simulink model "COSTEP"  (R2024b)
settings: Solver=FixedStepAuto  StartTime=0.0  StopTime=25  FixedStep=1/3600  RelTol=1e-3
model workspace (MAT data in the model file):
  AD : Simulink.Parameter (value not decoded)
  AG : Simulink.Parameter (value not decoded)
  AH : Simulink.Parameter (value not decoded)
  AV : Simulink.Parameter (value not decoded)
  AVP : Simulink.Parameter (value not decoded)
  BCHL : Simulink.Parameter (value not decoded)
  BCHV : Simulink.Parameter (value not decoded)
  BD : Simulink.Parameter (value not decoded)
  BDIST : Simulink.Parameter (value not decoded)
  BG : Simulink.Parameter (value not decoded)
  BH : Simulink.Parameter (value not decoded)
  BVP : Simulink.Parameter (value not decoded)
  CD : Simulink.Parameter (value not decoded)
  CDIST : Simulink.Parameter (value not decoded)
  CG : Simulink.Parameter (value not decoded)
  CH : Simulink.Parameter (value not decoded)
  CVP : Simulink.Parameter (value not decoded)
  DDIST : Simulink.Parameter (value not decoded)
  DIST_CONST : Simulink.Parameter (value not decoded)
  ISV : Simulink.Parameter (value not decoded)
  TLAST : Simulink.Parameter (value not decoded)
  TNEXT : Simulink.Parameter (value not decoded)
  XMW : Simulink.Parameter (value not decoded)
  XNS : Simulink.Parameter (value not decoded)
  XNS2 : Simulink.Parameter (value not decoded)
  XNS3 : Simulink.Parameter (value not decoded)
  XNSADD : Simulink.Parameter (value not decoded)
  XNSE : Simulink.Parameter (value not decoded)
symbols that are objects in the model workspace (value not decoded): AD, AG, AH, AV, AVP, BD, BG, BH, BVP, CD, CG, CH, CVP, XMW, XNS, XNS2, XNS3, XNSE
undefined symbols (not defined in the file or in its folder): magnitude, msgbox, SETPT, XMEAS, XMV
libraries: mylib x381, dspindex x31
(part 9 of 12)

== system COSTEP/Stream Measurements/Subsystem6/Product stream/Temperature measurement in C ==
  XMEAS in celsius : Inport
  SMEAST : Outport
  wires:
  XMEAS in celsius/1 -> SMEAST/1  "SMEAST"

== system COSTEP/Stream Measurements/Subsystem6/Purge stream/Composition measurement mol% ==
  XMEAS : Inport
  Bus Creator : BusCreator  Inputs=8
  Bus Selector : BusSelector  OutputSignals=XMEAS(29),XMEAS(30),XMEAS(31),XMEAS(32),XMEAS(33),XMEAS(34),XMEAS(35),XMEAS(36)
  SMEASX(9) : Outport
  wires:
  Bus Selector/4 -> Bus Creator/4  "<XMEAS(32)>"
  Bus Selector/5 -> Bus Creator/5  "<XMEAS(33)>"
  Bus Selector/6 -> Bus Creator/6  "<XMEAS(34)>"
  Bus Selector/7 -> Bus Creator/7  "<XMEAS(35)>"
  Bus Selector/8 -> Bus Creator/8  "<XMEAS(36)>"
  Bus Selector/3 -> Bus Creator/3  "<XMEAS(31)>"
  XMEAS/1 -> Bus Selector/1
  Bus Selector/2 -> Bus Creator/2  "<XMEAS(30)>"
  Bus Selector/1 -> Bus Creator/1  "<XMEAS(29)>"
  Bus Creator/1 -> SMEASX(9)/1  "SMEASX"

== system COSTEP/Stream Measurements/Subsystem6/Purge stream/Flow measurement in kg//h ==
  XMEAS in kscmh : Inport
  XST : Inport  Port=2
  " " : Constant  Value=35.3145
  "  " : Constant  Value=0.359
  Convert from lb/h to kg/h : Constant  Value=0.454
  Product : Product  Inputs=3
  XMWS Molecular weight of Stream lb/lb-mol : Subsystem
  lb-mol/h : Product  Inputs=**/
  "SMEASF(9) " : Outport  VectorParamsAs1DForOutWhenUnconnected=off
  wires:
  " "/1 -> lb-mol/h/2
  "  "/1 -> lb-mol/h/3
  XMEAS in kscmh/1 -> lb-mol/h/1
  Convert from lb/h to kg/h/1 -> Product/3
  XST/1 -> XMWS Molecular weight of Stream lb/lb-mol/1(XST)
  lb-mol/h/1 -> Product/2
  XMWS Molecular weight of Stream lb/lb-mol/1(XMWS) -> Product/1
  Product/1 -> "SMEASF(9) "/1

== system COSTEP/Stream Measurements/Subsystem6/Purge stream/Pressure measurement in kPa ==
  XMNSE : Inport
  " kPa" : Constant  Value=101.325
  Add : Sum
  SMEASP(9) : Outport  VectorParamsAs1DForOutWhenUnconnected=off
  wires:
  Add/1 -> SMEASP(9)/1  "SMEASP"
  " kPa"/1 -> Add/1
  XMNSE/1 -> Add/2

== system COSTEP/Stream Measurements/Subsystem6/Purge stream/Temperature measurement in C ==
  XMEAS in celsius : Inport
  SMEAST(9) : Outport
  wires:
  XMEAS in celsius/1 -> SMEAST(9)/1  "SMEAST"

== system COSTEP/Stream Measurements/Subsystem6/RCIn/Flow measurement in kg//h ==
  XMNSE : Inport
  F in gpm : Inport  Port=2
  Add : Sum
  Product : Product
  Product1 : Product
  gpm to lb/h : Constant  Value=500.72
  kg/kmol : Constant  Value=18.02
  kmol : Constant  Value=0.45359237
  kmol/h : Product
  lb/h to lb-mol/h : Product  Inputs=*/
  lb/lb-mol : Constant  Value=18.02
  "SMEASF " : Outport  VectorParamsAs1DForOutWhenUnconnected=off
  wires:
  Add/1 -> "SMEASF "/1  "SMEASF"
  Product/1 -> Add/1
  XMNSE/1 -> Add/2
  Product1/1 -> lb/h to lb-mol/h/1
  lb/lb-mol/1 -> lb/h to lb-mol/h/2
  lb/h to lb-mol/h/1 -> kmol/h/2
  gpm to lb/h/1 -> Product1/2
  F in gpm/1 -> Product1/1
  kmol/1 -> kmol/h/1
  kmol/h/1 -> Product/1
  kg/kmol/1 -> Product/2

== system COSTEP/Stream Measurements/Subsystem6/RCIn/Pressure measurement in kPa ==
  XMNSE : Inport
  TC : Inport  Port=2
  A Antoine Coefficient A : Constant  Value=11.6834
  Add : Sum
  Add1 : Sum
  Add2 : Sum  Inputs=+-
  B Antoine Coefficient B : Constant  Value=3816.44
  C Antoine Coefficient C : Constant  Value=-46.13
  Divide : Product  Inputs=*/
  Divide1 : Product  Inputs=**
  Math Function : Math  SignedPower=on
  Temperature in Kelvin K : Sum
  To Convert bar to kPa : Constant  Value=100
  To Convert °C to K : Constant  Value=273.15
  SMEASP : Outport  VectorParamsAs1DForOutWhenUnconnected=off
  wires:
  Add/1 -> SMEASP/1  "SMEASP"
  XMNSE/1 -> Add/2
  To Convert °C to K/1 -> Temperature in Kelvin K/2
  TC/1 -> Temperature in Kelvin K/1
  C Antoine Coefficient C/1 -> Add1/1
  Divide/1 -> Add2/2
  B Antoine Coefficient B/1 -> Divide/1
  Add1/1 -> Divide/2
  Math Function/1 -> Divide1/1
  A Antoine Coefficient A/1 -> Add2/1
  Add2/1 -> Math Function/1
  To Convert bar to kPa/1 -> Divide1/2
  Temperature in Kelvin K/1 -> Add1/2
  Divide1/1 -> Add/1

== system COSTEP/Stream Measurements/Subsystem6/RCIn/Temperature measurement in C ==
  T in celsius : Inport
  XMNSE : Inport  Port=2
  Add : Sum
  SMEAST : Outport
  wires:
  T in celsius/1 -> Add/1
  Add/1 -> SMEAST/1  "SMEAST"
  XMNSE/1 -> Add/2

== system COSTEP/Stream Measurements/Subsystem6/RCOut/Pressure measurement in kPa ==
  XMNSE : Inport
  TC : Inport  Port=2
  A Antoine Coefficient A : Constant  Value=11.6834
  Add : Sum
  Add1 : Sum
  Add2 : Sum  Inputs=+-
  B Antoine Coefficient B : Constant  Value=3816.44
  C Antoine Coefficient C : Constant  Value=-46.13
  Divide : Product  Inputs=*/
  Divide1 : Product  Inputs=**
  Math Function : Math  SignedPower=on
  Temperature in Kelvin K : Sum
  To Convert bar to kPa : Constant  Value=100
  To Convert °C to K : Constant  Value=273.15
  SMEASP : Outport  VectorParamsAs1DForOutWhenUnconnected=off
  wires:
  Add/1 -> SMEASP/1  "SMEASP"
  XMNSE/1 -> Add/2
  To Convert °C to K/1 -> Temperature in Kelvin K/2
  TC/1 -> Temperature in Kelvin K/1
  C Antoine Coefficient C/1 -> Add1/1
  Divide/1 -> Add2/2
  B Antoine Coefficient B/1 -> Divide/1
  Add1/1 -> Divide/2
  Math Function/1 -> Divide1/1
  A Antoine Coefficient A/1 -> Add2/1
  Add2/1 -> Math Function/1
  To Convert bar to kPa/1 -> Divide1/2
  Temperature in Kelvin K/1 -> Add1/2
  Divide1/1 -> Add/1

== system COSTEP/Stream Measurements/Subsystem6/RCOut/Temperature measurement in C ==
  T in celsius : Inport
  XMNSE : Inport  Port=2
  Add : Sum
  SMEAST : Outport
  wires:
  T in celsius/1 -> Add/1
  Add/1 -> SMEAST/1  "SMEAST"
  XMNSE/1 -> Add/2

== system COSTEP/Stream Measurements/Subsystem6/Reactor feed stream/Composition measurement mol% ==
  XST : Inport
  XMNSE : Inport  Port=2
  XMEAS : Inport  Port=3
  Bus Creator : BusCreator  Inputs=8
  Subsystem : Subsystem
  SMEASX(6) : Outport
  wires:
  Subsystem/4(SMEASXD) -> Bus Creator/4  "SMEASXD(6)"
  Subsystem/5(SMEASXE) -> Bus Creator/5  "SMEASXE(6)"
  Subsystem/6(SMEASXF) -> Bus Creator/6  "SMEASXF(6)"
  Subsystem/7(SMEASXG) -> Bus Creator/7  "SMEASXG(6)"
  Subsystem/8(SMEASXH) -> Bus Creator/8  "SMEASXH(6)"
  Subsystem/3(SMEASXC) -> Bus Creator/3  "SMEASXC(6)"
  XST/1 -> Subsystem/1(XST)
  Subsystem/2(SMEASXB) -> Bus Creator/2  "SMEASXB(6)"
  Subsystem/1(SMEASXA) -> Bus Creator/1  "SMEASXA(6)"
  Bus Creator/1 -> SMEASX(6)/1  "SMEASX(6)"
  XMNSE/1 -> Subsystem/2(XMNSE)
  XMEAS/1 -> Subsystem/3(XMEAS)

== system COSTEP/Stream Measurements/Subsystem6/Reactor feed stream/Flow measurement in kg//h ==
  XMEAS in kscmh : Inport
  XST : Inport  Port=2
  " " : Constant  Value=35.3145
  "  " : Constant  Value=0.359
  Convert from lb/h to kg/h : Constant  Value=0.454
  Product : Product  Inputs=3
  XMWS Molecular weight of Stream lb/lb-mol : Subsystem
  lb-mol/h : Product  Inputs=**/
  "SMEASF " : Outport  VectorParamsAs1DForOutWhenUnconnected=off
  wires:
  " "/1 -> lb-mol/h/2
  "  "/1 -> lb-mol/h/3
  XMEAS in kscmh/1 -> lb-mol/h/1
  Convert from lb/h to kg/h/1 -> Product/3
  XST/1 -> XMWS Molecular weight of Stream lb/lb-mol/1(XST)
  lb-mol/h/1 -> Product/2
  XMWS Molecular weight of Stream lb/lb-mol/1(XMWS) -> Product/1
  Product/1 -> "SMEASF "/1

== system COSTEP/Stream Measurements/Subsystem6/Reactor feed stream/Pressure measurement in kPa ==
  XMEAS in kPa gauge : Inport
  " kPa" : Constant  Value=101.325
  Add : Sum
  SMEASP : Outport  VectorParamsAs1DForOutWhenUnconnected=off
  wires:
  Add/1 -> SMEASP/1  "SMEASP"
  " kPa"/1 -> Add/2
  XMEAS in kPa gauge/1 -> Add/1

== system COSTEP/Stream Measurements/Subsystem6/Reactor feed stream/Temperature measurement in C ==
  T in celsius : Inport
  XMNSE : Inport  Port=2
  Add : Sum
  SMEAST : Outport
  wires:
  T in celsius/1 -> Add/1
  Add/1 -> SMEAST/1  "SMEAST"
  XMNSE/1 -> Add/2

== system COSTEP/Stream Measurements/Subsystem6/Reactor product stream/Composition measurement mol% ==
  XST : Inport
  XMNSE : Inport  Port=2
  Bus Creator : BusCreator  Inputs=8
  Subsystem : Subsystem
  SMEASX(7) : Outport
  wires:
  Subsystem/4(SMEASXD(7)) -> Bus Creator/4  "SMEASXD(7)"
  Subsystem/5(SMEASXE(7)) -> Bus Creator/5  "SMEASXE(7)"
  Subsystem/6(SMEASXF(7)) -> Bus Creator/6  "SMEASXF(7)"
  Subsystem/7(SMEASXG(7)) -> Bus Creator/7  "SMEASXG(7)"
  Subsystem/8(SMEASXH(7)) -> Bus Creator/8  "SMEASXH(7)"
  Subsystem/3(SMEASXC(7)) -> Bus Creator/3  "SMEASXC(7)"
  XST/1 -> Subsystem/1(XST)
  Subsystem/2(SMEASXB(7)) -> Bus Creator/2  "SMEASXB(7)"
  Subsystem/1(SMEASXA(7)) -> Bus Creator/1  "SMEASXA(7)"
  Bus Creator/1 -> SMEASX(7)/1  "SMEASX"
  XMNSE/1 -> Subsystem/2(XMNSE)

== system COSTEP/Stream Measurements/Subsystem6/Reactor product stream/Flow measurement in kg//h ==
  XST : Inport
  XMNSE : Inport  Port=2
  F in lb-mol/h : Inport  Port=3
  Add : Sum
  Convert from lb/h to kg/h : Constant  Value=0.454
  Product : Product  Inputs=3
  XMWS Molecular weight of Stream lb/lb-mol : Subsystem
  "SMEASF(7) " : Outport  VectorParamsAs1DForOutWhenUnconnected=off
  wires:
  Convert from lb/h to kg/h/1 -> Product/3
  Add/1 -> "SMEASF(7) "/1  "SMEASF(7)"
  Product/1 -> Add/1
  XST/1 -> XMWS Molecular weight of Stream lb/lb-mol/1(XST)
  XMWS Molecular weight of Stream lb/lb-mol/1(XMWS) -> Product/1
  XMNSE/1 -> Add/2
  F in lb-mol/h/1 -> Product/2

== system COSTEP/Stream Measurements/Subsystem6/Reactor product stream/Pressure measurement in kPa ==
  XMEAS in kPa gauge : Inport
  " kPa" : Constant  Value=101.325
  Add : Sum
  SMEASP(7) : Outport  VectorParamsAs1DForOutWhenUnconnected=off
  wires:
  Add/1 -> SMEASP(7)/1  "SMEASP"
  " kPa"/1 -> Add/2
  XMEAS in kPa gauge/1 -> Add/1

== system COSTEP/Stream Measurements/Subsystem6/Reactor product stream/Temperature measurement in C ==
  XMEAS in celsius : Inport
  SMEAST(7) : Outport
  wires:
  XMEAS in celsius/1 -> SMEAST(7)/1  "SMEAST"

== system COSTEP/Stream Measurements/Subsystem6/Separator product stream/Composition measurement mol% ==
  XST : Inport
  XMNSE : Inport  Port=2
  Bus Creator : BusCreator  Inputs=8
  Subsystem : Subsystem
  SMEASX : Outport
  wires:
  Subsystem/4(SMEASXD) -> Bus Creator/4  "SMEASXD"
  Subsystem/5(SMEASXE) -> Bus Creator/5  "SMEASXE"
  Subsystem/6(SMEASXF) -> Bus Creator/6  "SMEASXF"
  Subsystem/7(SMEASXG) -> Bus Creator/7  "SMEASXG"
  Subsystem/8(SMEASXH) -> Bus Creator/8  "SMEASXH"
  Subsystem/3(SMEASXC) -> Bus Creator/3  "SMEASXC"
  XST/1 -> Subsystem/1(XST)
  Subsystem/2(SMEASXB) -> Bus Creator/2  "SMEASXB"
  Subsystem/1(SMEASXA) -> Bus Creator/1  "SMEASXA"
  Bus Creator/1 -> SMEASX/1  "SMEASX"
  XMNSE/1 -> Subsystem/2(XMNSE)

== system COSTEP/Stream Measurements/Subsystem6/Separator product stream/Flow measurement in kg//h ==
  XMEAS in kscmh : Inport
  XST : Inport  Port=2
  XMEAS in kscmh1 : Inport  Port=3
  Add : Sum
  Subsystem : Subsystem
  Subsystem1 : Subsystem
  "SMEASF " : Outport  VectorParamsAs1DForOutWhenUnconnected=off
  wires:
  XST/1 -> Subsystem1/1(XST), Subsystem/1(XST)
  XMEAS in kscmh/1 -> Subsystem/2(XMEAS)
  Subsystem/1(SMEAS F) -> Add/1
  Add/1 -> "SMEASF "/1
  Subsystem1/1(SMEAS F) -> Add/2
  XMEAS in kscmh1/1 -> Subsystem1/2(XMEAS)

== system COSTEP/Stream Measurements/Subsystem6/Separator product stream/Pressure measurement in kPa ==
  XMEAS in kPa gauge : Inport
  " kPa" : Constant  Value=101.325
  Add : Sum
  SMEASP : Outport  VectorParamsAs1DForOutWhenUnconnected=off
  wires:
  Add/1 -> SMEASP/1  "SMEASP"
  " kPa"/1 -> Add/2
  XMEAS in kPa gauge/1 -> Add/1

== system COSTEP/Stream Measurements/Subsystem6/Separator product stream/Temperature measurement in C ==
  XMEAS in celsius : Inport
  SMEAST : Outport
  wires:
  XMEAS in celsius/1 -> SMEAST/1  "SMEAST"

== system COSTEP/Stream Measurements/Subsystem6/Separator recycle stream (after compressor)/Composition measurement mol% ==
  XST : Inport
  XMNSE : Inport  Port=2
  Bus Creator : BusCreator  Inputs=8
  Subsystem : Subsystem
  SMEASX(8) : Outport
  wires:
  Subsystem/4(SMEASXD) -> Bus Creator/4  "SMEASXD(8)"
  Subsystem/5(SMEASXE) -> Bus Creator/5  "SMEASXE(8)"
  Subsystem/6(SMEASXF) -> Bus Creator/6  "SMEASXF(8)"
  Subsystem/7(SMEASXG) -> Bus Creator/7  "SMEASXG(8)"
  Subsystem/8(SMEASXH) -> Bus Creator/8  "SMEASXH(8)"
  Subsystem/3(SMEASXC) -> Bus Creator/3  "SMEASXC(8)"
  XST/1 -> Subsystem/1(XST)
  Subsystem/2(SMEASXB) -> Bus Creator/2  "SMEASXB(8)"
  Subsystem/1(SMEASXA) -> Bus Creator/1  "SMEASXA(8)"
  Bus Creator/1 -> SMEASX(8)/1  "SMEASX"
  XMNSE/1 -> Subsystem/2(XMNSE)

== system COSTEP/Stream Measurements/Subsystem6/Separator recycle stream (after compressor)/Flow measurement in kg//h ==
  XMEAS in kscmh : Inport
  XST : Inport  Port=2
  " " : Constant  Value=35.3145
  "  " : Constant  Value=0.359
  Convert from lb/h to kg/h : Constant  Value=0.454
  Product : Product  Inputs=3
  XMWS Molecular weight of Stream lb/lb-mol : Subsystem
  lb-mol/h : Product  Inputs=**/
  "SMEASF(8) " : Outport  VectorParamsAs1DForOutWhenUnconnected=off
  wires:
  " "/1 -> lb-mol/h/2
  "  "/1 -> lb-mol/h/3
  XMEAS in kscmh/1 -> lb-mol/h/1
  Convert from lb/h to kg/h/1 -> Product/3
  XST/1 -> XMWS Molecular weight of Stream lb/lb-mol/1(XST)
  lb-mol/h/1 -> Product/2
  XMWS Molecular weight of Stream lb/lb-mol/1(XMWS) -> Product/1
  Product/1 -> "SMEASF(8) "/1

== system COSTEP/Stream Measurements/Subsystem6/Separator recycle stream (after compressor)/Pressure measurement in kPa ==
  XMEAS in kPa gauge : Inport
  " kPa" : Constant  Value=101.325
  Add : Sum
  SMEASP(8) : Outport  VectorParamsAs1DForOutWhenUnconnected=off
  wires:
  Add/1 -> SMEASP(8)/1  "SMEASP"
  " kPa"/1 -> Add/2
  XMEAS in kPa gauge/1 -> Add/1

== system COSTEP/Stream Measurements/Subsystem6/Separator recycle stream (after compressor)/Temperature measurement in C ==
  HST(9) : Inport
  XST : Inport  Port=2
  ITY : Inport  Port=3
  "TST(9) Temperature of Stream °C " : Subsystem
  SMEAST(8) : Outport
  wires:
  "TST(9) Temperature of Stream °C "/1(TST(9)) -> SMEAST(8)/1  "SMEAST"
  HST(9)/1 -> "TST(9) Temperature of Stream °C "/1(HST)
  XST/1 -> "TST(9) Temperature of Stream °C "/2(XLR)
  ITY/1 -> "TST(9) Temperature of Stream °C "/3(ITY)

== system COSTEP/Stream Measurements/Subsystem6/Separator recycle stream (before compressor)/Composition measurement mol% ==
  XST : Inport
  XMNSE : Inport  Port=2
  Bus Creator : BusCreator  Inputs=8
  Subsystem : Subsystem
  SMEASX : Outport
  wires:
  Subsystem/4(SMEASXD) -> Bus Creator/4  "SMEASXD"
  Subsystem/5(SMEASXE) -> Bus Creator/5  "SMEASXE"
  Subsystem/6(SMEASXF) -> Bus Creator/6  "SMEASXF"
  Subsystem/7(SMEASXG) -> Bus Creator/7  "SMEASXG"
  Subsystem/8(SMEASXH) -> Bus Creator/8  "SMEASXH"
  Subsystem/3(SMEASXC) -> Bus Creator/3  "SMEASXC"
  XST/1 -> Subsystem/1(XST)
  Subsystem/2(SMEASXB) -> Bus Creator/2  "SMEASXB"
  Subsystem/1(SMEASXA) -> Bus Creator/1  "SMEASXA"
  Bus Creator/1 -> SMEASX/1  "SMEASX"
  XMNSE/1 -> Subsystem/2(XMNSE)

== system COSTEP/Stream Measurements/Subsystem6/Separator recycle stream (before compressor)/Flow measurement in kg//h ==
  XMEAS in kscmh : Inport
  XST : Inport  Port=2
  " " : Constant  Value=35.3145
  "  " : Constant  Value=0.359
  Convert from lb/h to kg/h : Constant  Value=0.454
  Product : Product  Inputs=3
  XMWS Molecular weight of Stream lb/lb-mol : Subsystem
  lb-mol/h : Product  Inputs=**/
  "SMEASF " : Outport  VectorParamsAs1DForOutWhenUnconnected=off
  wires:
  " "/1 -> lb-mol/h/2
  "  "/1 -> lb-mol/h/3
  XMEAS in kscmh/1 -> lb-mol/h/1
  Convert from lb/h to kg/h/1 -> Product/3
  XST/1 -> XMWS Molecular weight of Stream lb/lb-mol/1(XST)
  lb-mol/h/1 -> Product/2
  XMWS Molecular weight of Stream lb/lb-mol/1(XMWS) -> Product/1
  Product/1 -> "SMEASF "/1

== system COSTEP/Stream Measurements/Subsystem6/Separator recycle stream (before compressor)/Pressure measurement in kPa ==
  XMEAS in kPa gauge : Inport
  " kPa" : Constant  Value=101.325
  Add : Sum
  SMEASP : Outport  VectorParamsAs1DForOutWhenUnconnected=off
  wires:
  Add/1 -> SMEASP/1  "SMEASP"
  " kPa"/1 -> Add/2
  XMEAS in kPa gauge/1 -> Add/1

== system COSTEP/Stream Measurements/Subsystem6/Separator recycle stream (before compressor)/Temperature measurement in C ==
  XMEAS in celsius : Inport
  SMEAST : Outport
  wires:
  XMEAS in celsius/1 -> SMEAST/1  "SMEAST"

== system COSTEP/Stream Measurements/Subsystem6/Separator underflow stream/Composition measurement mol% ==
  XST : Inport
  XMNSE : Inport  Port=2
  Bus Creator : BusCreator  Inputs=5
  Subsystem : Subsystem
  SMEASX : Outport
  wires:
  Subsystem/1(SMEASXD) -> Bus Creator/1  "SMEASXD"
  Subsystem/2(SMEASXE) -> Bus Creator/2  "SMEASXE"
  Subsystem/3(SMEASXF) -> Bus Creator/3  "SMEASXF"
  Subsystem/4(SMEASXG) -> Bus Creator/4  "SMEASXG"
  Subsystem/5(SMEASXH) -> Bus Creator/5  "SMEASXH"
  XST/1 -> Subsystem/1(XST)
  Bus Creator/1 -> SMEASX/1  "SMEASX"
  XMNSE/1 -> Subsystem/2(XMNSE)

== system COSTEP/Stream Measurements/Subsystem6/Separator underflow stream/Flow measurement in kg//h ==
  XMEAS in m^3/h : Inport
  XST : Inport  Port=2
  "       " : Constant  Value=35.3145
  Convert from lb/h to kg/h : Constant  Value=0.454
  XMWS Molecular weight of Stream lb/lb-mol : Subsystem
  kg/h : Product  Inputs=3
  lb-mol/h : Product  Inputs=***
  "SMEASF " : Outport  VectorParamsAs1DForOutWhenUnconnected=off
  wires:
  lb-mol/h/1 -> kg/h/2
  [DLS] -> lb-mol/h/2
  "       "/1 -> lb-mol/h/3
  XMEAS in m^3/h/1 -> lb-mol/h/1
  XMWS Molecular weight of Stream lb/lb-mol/1(XMWS) -> kg/h/1
  Convert from lb/h to kg/h/1 -> kg/h/3
  kg/h/1 -> "SMEASF "/1
  XST/1 -> XMWS Molecular weight of Stream lb/lb-mol/1(XST)

== system COSTEP/Stream Measurements/Subsystem6/Separator underflow stream/Pressure measurement in kPa ==
  "P in mm Hg " : Inport
  XMNSE : Inport  Port=2
  " kPa" : Constant  Value=101.325
  " mm Hg   " : Constant  Value=760
  Add : Sum
  Pressure conversion kPa : Product  Inputs=*/*
  SMEASP : Outport  VectorParamsAs1DForOutWhenUnconnected=off
  wires:
  "P in mm Hg "/1 -> Pressure conversion kPa/1
  " kPa"/1 -> Pressure conversion kPa/3
  " mm Hg   "/1 -> Pressure conversion kPa/2
  Pressure conversion kPa/1 -> Add/1
  Add/1 -> SMEASP/1  "SMEASP"
  XMNSE/1 -> Add/2

== system COSTEP/Stream Measurements/Subsystem6/Separator underflow stream/Temperature measurement in C ==
  XMEAS in celsius : Inport
  SMEAST : Outport
  wires:
  XMEAS in celsius/1 -> SMEAST/1  "SMEAST"

== system COSTEP/Stream Measurements/Subsystem6/Stripper recycle stream/Composition measurement mol% ==
  XST : Inport
  XMNSE : Inport  Port=2
  Bus Creator : BusCreator  Inputs=8
  Subsystem : Subsystem
  SMEASX(5) : Outport
  wires:
  Subsystem/4(SMEASXD) -> Bus Creator/4  "SMEASXD(5)"
  Subsystem/5(SMEASXE) -> Bus Creator/5  "SMEASXE(5)"
  Subsystem/6(SMEASXF) -> Bus Creator/6  "SMEASXF(5)"
  Subsystem/7(SMEASXG) -> Bus Creator/7  "SMEASXG(5)"
  Subsystem/8(SMEASXH) -> Bus Creator/8  "SMEASXH(5)"
  Subsystem/3(SMEASXC) -> Bus Creator/3  "SMEASXC(5)"
  XST/1 -> Subsystem/1(XST)
  Subsystem/2(SMEASXB) -> Bus Creator/2  "SMEASXB(5)"
  Subsystem/1(SMEASXA) -> Bus Creator/1  "SMEASXA(5)"
  Bus Creator/1 -> SMEASX(5)/1  "SMEASX(5)"
  XMNSE/1 -> Subsystem/2(XMNSE)

== system COSTEP/Stream Measurements/Subsystem6/Stripper recycle stream/Flow measurement in kg//h ==
  XST : Inport
  XMNSE : Inport  Port=2
  F in lb-mol/h : Inport  Port=3
  Add : Sum
  Convert from lb/h to kg/h : Constant  Value=0.454
  Product : Product  Inputs=3
  XMWS Molecular weight of Stream lb/lb-mol : Subsystem
  "SMEASF(5) " : Outport  VectorParamsAs1DForOutWhenUnconnected=off
  wires:
  Convert from lb/h to kg/h/1 -> Product/3
  Add/1 -> "SMEASF(5) "/1  "SMEASF(5)"
  Product/1 -> Add/1
  XST/1 -> XMWS Molecular weight of Stream lb/lb-mol/1(XST)
  XMWS Molecular weight of Stream lb/lb-mol/1(XMWS) -> Product/1
  XMNSE/1 -> Add/2
  F in lb-mol/h/1 -> Product/2

== system COSTEP/Stream Measurements/Subsystem6/Stripper recycle stream/Pressure measurement in kPa ==
  XMEAS in kPa gauge : Inport
  " kPa" : Constant  Value=101.325
  Add : Sum
  SMEASP(5) : Outport  VectorParamsAs1DForOutWhenUnconnected=off
  wires:
  Add/1 -> SMEASP(5)/1  "SMEASP(5)"
  " kPa"/1 -> Add/2
  XMEAS in kPa gauge/1 -> Add/1

== system COSTEP/Stream Measurements/Subsystem6/Stripper recycle stream/Temperature measurement in C ==
  T in celsius : Inport
  XMNSE : Inport  Port=2
  Add : Sum
  SMEAST(5) : Outport
  wires:
  T in celsius/1 -> Add/1
  Add/1 -> SMEAST(5)/1  "SMEAST"
  XMNSE/1 -> Add/2

== system COSTEP/Stripper/Split Fractions/Split fraction/If Action Subsystem ==
  In1 : Inport
  Action Port : ActionPort  ActionPortLabel=if(u1 >0.1)
  Out1 : Outport  VectorParamsAs1DForOutWhenUnconnected=off
  wires:
  In1/1 -> Out1/1

== system COSTEP/Stripper/Split Fractions/Split fraction/If Action Subsystem1 ==
  In1 : Inport
  Action Port : ActionPort  ActionPortLabel=if(u1 >170)
  Out1 : Outport  VectorParamsAs1DForOutWhenUnconnected=off
  wires:
  In1/1 -> Out1/1

== system COSTEP/Stripper/Split Fractions/Split fraction/If Action Subsystem2 ==
  In1 : Inport
  Action Port : ActionPort  ActionPortLabel=elseif(u1<5.292)
  Out1 : Outport  VectorParamsAs1DForOutWhenUnconnected=off
  wires:
  In1/1 -> Out1/1

== system COSTEP/Stripper/Split Fractions/Split fraction/If Action Subsystem3 ==
  In1 : Inport
  Action Port : ActionPort  ActionPortLabel=else
  Out1 : Outport  VectorParamsAs1DForOutWhenUnconnected=off
  wires:
  In1/1 -> Out1/1

== system COSTEP/Stripper/Split Fractions/Split fraction/If Action Subsystem4 ==
  In1 : Inport
  Action Port : ActionPort  ActionPortLabel=else
  Out1 : Outport  VectorParamsAs1DForOutWhenUnconnected=off
  wires:
  In1/1 -> Out1/1

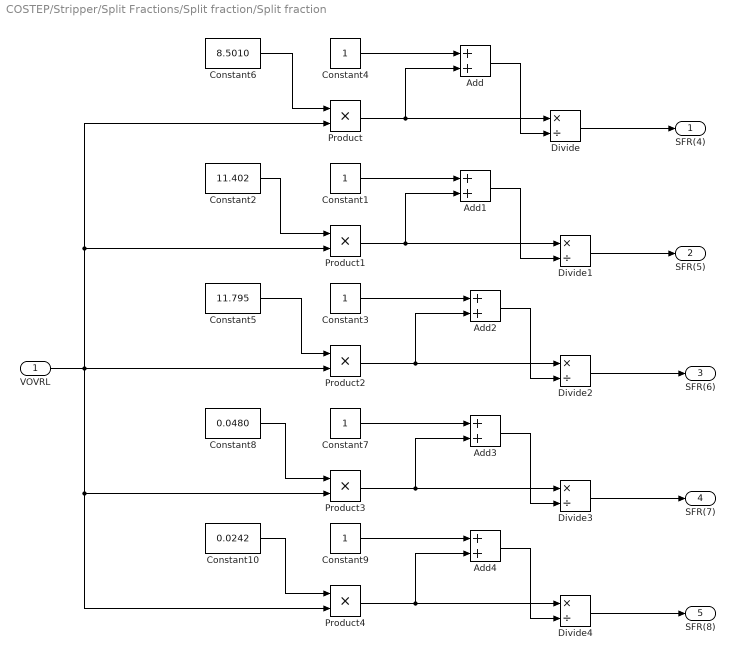
== system COSTEP/Stripper/Split Fractions/Split fraction/Split fraction ==
  VOVRL : Inport
  Add{,1..4} (5 alike) : Sum
  Constant{1,3..4,7,9} (5 alike) : Constant
  Constant10 : Constant  Value=0.0242
  Constant2 : Constant  Value=11.402
  Constant5 : Constant  Value=11.795
  Constant6 : Constant  Value=8.5010
  Constant8 : Constant  Value=0.0480
  Divide{,1..4} (5 alike) : Product  Inputs=*/
  Product{,1..4} (5 alike) : Product
  SFR(4) : Outport  PortDimensions=1  VectorParamsAs1DForOutWhenUnconnected=off
  SFR(5) : Outport  Port=2  PortDimensions=1  VectorParamsAs1DForOutWhenUnconnected=off
  SFR(6) : Outport  Port=3  PortDimensions=1  VectorParamsAs1DForOutWhenUnconnected=off
  SFR(7) : Outport  Port=4  PortDimensions=1  VectorParamsAs1DForOutWhenUnconnected=off
  SFR(8) : Outport  Port=5  PortDimensions=1  VectorParamsAs1DForOutWhenUnconnected=off
  wires:
  Add/1 -> Divide/2
  Product/1 -> Divide/1, Add/2
  Constant4/1 -> Add/1
  Constant6/1 -> Product/1
  Divide/1 -> SFR(4)/1
  Product1/1 -> Divide1/1, Add1/2
  Add1/1 -> Divide1/2
  Constant1/1 -> Add1/1
  Constant2/1 -> Product1/1
  Divide1/1 -> SFR(5)/1
  Divide2/1 -> SFR(6)/1
  Product2/1 -> Divide2/1, Add2/2
  Add2/1 -> Divide2/2
  Constant3/1 -> Add2/1
  Constant5/1 -> Product2/1
  Divide3/1 -> SFR(7)/1
  Product3/1 -> Divide3/1, Add3/2
  Add3/1 -> Divide3/2
  Constant7/1 -> Add3/1
  Constant8/1 -> Product3/1
  Divide4/1 -> SFR(8)/1
  Product4/1 -> Divide4/1, Add4/2
  VOVRL/1 -> Product/2, Product1/2, Product4/2, Product3/2, Product2/2
  Add4/1 -> Divide4/2
  Constant9/1 -> Add4/1
  Constant10/1 -> Product4/1

== system COSTEP/Stripper/Volume of Stripper/DLC Molar Density of Liquids in Stripper lb-mol//ft³    /DLC Molar Density of Liquids in Stripper lb-mol//ft³  ==
  X : Inport
  T : Inport  Port=2
  "  " : Constant
  "    " : Product  Inputs=*/
  AD(I) : Constant  Value=AD
  Add2 : Sum
  BD(I) : Constant  Value=BD
  CD(I) : Constant  Value=CD
  Constant : Constant  Value=XMW
  Liquid Density of Components lb/ft³ : Sum
  Product : Product
  Product1 : Product
  Product2 : Product
  Sum of Elements : Sum  Inputs=+
  V Molar Volume of Components ft³/lb-mol : Product  Inputs=*/
  "R " : Outport  VectorParamsAs1DForOutWhenUnconnected=off
  wires:
  Liquid Density of Components lb/ft³/1 -> V Molar Volume of Components ft³/lb-mol/2
  Product1/1 -> Liquid Density of Components lb/ft³/2
  T/1 -> Product1/2, Product/2
  "  "/1 -> "    "/1
  AD(I)/1 -> Liquid Density of Components lb/ft³/1
  Add2/1 -> Product1/1
  V Molar Volume of Components ft³/lb-mol/1 -> Sum of Elements/1
  CD(I)/1 -> Product/1
  Product2/1 -> V Molar Volume of Components ft³/lb-mol/1
  BD(I)/1 -> Add2/1
  Product/1 -> Add2/2
  "    "/1 -> "R "/1
  X/1 -> Product2/1
  Sum of Elements/1 -> "    "/2
  Constant/1 -> Product2/2

== system COSTEP/Control Mode/Braatz/ /CONTROL 14/PI Control Setpoint Velocity form ==
  Setpoint : Inport
  Measurement : Inport  Port=2
  Gain : Gain  Gain=H/100
  Subsystem : Subsystem  mask{Kc=Kc, Ti=Ti, Ts=Ts, HS=HS}
      mask prompts: Kc "Controller Gain - Kc"; Ti "Integral Time - Ti"; Ts "Sampling Interval - Ts"; HS "High limit of setpoint"
      mask DialogControl DescGroupVar Prompt: Control Parameters
  Sum : Sum  Inputs=|++  SaturateOnIntegerOverflow=on
  Unit Delay : UnitDelay  InitialCondition=X_0  SampleTime=Ts
  Output : Outport
  wires:
  Gain/1 -> Sum/1
  Subsystem/1(Delta Output) -> Gain/1
  Measurement/1 -> Subsystem/2(Measurement)
  Setpoint/1 -> Subsystem/1(Setpoint)
  Sum/1 -> Unit Delay/1, Output/1
  Unit Delay/1 -> Sum/2

== system COSTEP/Control Mode/Braatz/ 10/CONTROL 6/P Control Velocity form ==
  Setpoint : Inport
  Measurement : Inport  Port=2
  XMEAS : Inport  Port=3
  Pressure limits : Subsystem
      mask Display: color('Blue'),disp('Pressure limits'),
  Subsystem : Subsystem  mask{Kc=Kc, Ts=Ts, H=H}
      mask prompts: Kc "Controller Gain - Kc"; Ts "Sampling Interval - Ts"; H "High limit of measurement"
      mask DialogControl DescGroupVar Prompt: Control Parameters
  Sum : Sum  Inputs=|++  SaturateOnIntegerOverflow=on
  Unit Delay : UnitDelay  InitialCondition=X_0  SampleTime=Ts
  Output : Outport
  wires:
  Unit Delay/1 -> Output/1, Sum/2
  Sum/1 -> Pressure limits/1("XMV(6) ")
  Setpoint/1 -> Subsystem/1(Setpoint)
  Pressure limits/1(XMV(6)) -> Unit Delay/1
  Subsystem/1(Delta Output) -> Sum/1
  Measurement/1 -> Subsystem/2(Measurement)
  XMEAS/1 -> Pressure limits/2(XMEAS)

== system COSTEP/Random number generator/Stream Measurements SMEAS Gas analysis1/Gas Analysis Delay/Subsystem/If Action Subsystem ==
  Action Port : ActionPort  ActionPortLabel=if(u1 == u2)
  Constant : Constant  Value=0
  Out1 : Outport  VectorParamsAs1DForOutWhenUnconnected=off
  wires:
  Constant/1 -> Out1/1

== system COSTEP/Random number generator/Stream Measurements SMEAS Gas analysis1/Gas Analysis Delay/Subsystem/If Action Subsystem1 ==
  In1 : Inport
  Action Port : ActionPort  ActionPortLabel=else
  Out1 : Outport  VectorParamsAs1DForOutWhenUnconnected=off
  wires:
  In1/1 -> Out1/1

== system COSTEP/Random number generator/Stream Measurements SMEAS Gas analysis1/If Action Subsystem3/Subsystem/Stream 1 ==
  G : Inport
  Bus Creator : BusCreator  Inputs=8
  Subsystem : Subsystem
  Stream 1 : Outport
  G_NEW : Outport  Port=2
  wires:
  Subsystem/4(XMNSED) -> Bus Creator/4
  Subsystem/1(XMNSEA) -> Bus Creator/1
  G/1 -> Subsystem/1(G)
  Subsystem/8(XMNSEH) -> Bus Creator/8
  Subsystem/3(XMNSEC) -> Bus Creator/3
  Subsystem/7(XMNSEG) -> Bus Creator/7
  Subsystem/9(G_NEW) -> G_NEW/1
  Subsystem/2(XMNSEB) -> Bus Creator/2
  Subsystem/5(XMNSEE) -> Bus Creator/5
  Subsystem/6(XMNSEF) -> Bus Creator/6
  Bus Creator/1 -> Stream 1/1  "Stream 1"

== system COSTEP/Random number generator/Stream Measurements SMEAS Gas analysis1/If Action Subsystem3/Subsystem/Stream 13 ==
  G : Inport
  Bus Creator : BusCreator  Inputs=8
  Subsystem : Subsystem
  Stream 13 : Outport
  G_NEW : Outport  Port=2
  wires:
  Subsystem/4(XMNSED) -> Bus Creator/4
  Subsystem/1(XMNSEA) -> Bus Creator/1
  G/1 -> Subsystem/1(G)
  Subsystem/8(XMNSEH) -> Bus Creator/8
  Subsystem/3(XMNSEC) -> Bus Creator/3
  Subsystem/7(XMNSEG) -> Bus Creator/7
  Subsystem/9(G_NEW) -> G_NEW/1
  Subsystem/2(XMNSEB) -> Bus Creator/2
  Subsystem/5(XMNSEE) -> Bus Creator/5
  Subsystem/6(XMNSEF) -> Bus Creator/6
  Bus Creator/1 -> Stream 13/1  "Stream 13"

== system COSTEP/Random number generator/Stream Measurements SMEAS Gas analysis1/If Action Subsystem3/Subsystem/Stream 2 ==
  G : Inport
  Bus Creator : BusCreator  Inputs=8
  Subsystem : Subsystem
  Stream 2 : Outport
  G_NEW : Outport  Port=2
  wires:
  Subsystem/4(XMNSED) -> Bus Creator/4
  Subsystem/1(XMNSEA) -> Bus Creator/1
  G/1 -> Subsystem/1(G)
  Subsystem/8(XMNSEH) -> Bus Creator/8
  Subsystem/3(XMNSEC) -> Bus Creator/3
  Subsystem/7(XMNSEG) -> Bus Creator/7
  Subsystem/9(G_NEW) -> G_NEW/1
  Subsystem/2(XMNSEB) -> Bus Creator/2
  Subsystem/5(XMNSEE) -> Bus Creator/5
  Subsystem/6(XMNSEF) -> Bus Creator/6
  Bus Creator/1 -> Stream 2/1  "Stream 2"

== system COSTEP/Random number generator/Stream Measurements SMEAS Gas analysis1/If Action Subsystem3/Subsystem/Stream 3 ==
  G : Inport
  Bus Creator : BusCreator  Inputs=8
  Subsystem : Subsystem
  Stream 3 : Outport
  G_NEW : Outport  Port=2
  wires:
  Subsystem/4(XMNSED) -> Bus Creator/4
  Subsystem/1(XMNSEA) -> Bus Creator/1
  G/1 -> Subsystem/1(G)
  Subsystem/8(XMNSEH) -> Bus Creator/8
  Subsystem/3(XMNSEC) -> Bus Creator/3
  Subsystem/7(XMNSEG) -> Bus Creator/7
  Subsystem/9(G_NEW) -> G_NEW/1
  Subsystem/2(XMNSEB) -> Bus Creator/2
  Subsystem/5(XMNSEE) -> Bus Creator/5
  Subsystem/6(XMNSEF) -> Bus Creator/6
  Bus Creator/1 -> Stream 3/1  "Stream 3"

== system COSTEP/Random number generator/Stream Measurements SMEAS Gas analysis1/If Action Subsystem3/Subsystem/Stream 4 ==
  G : Inport
  Bus Creator : BusCreator  Inputs=8
  Subsystem : Subsystem
  Stream 4 : Outport
  G_NEW : Outport  Port=2
  wires:
  Subsystem/4(XMNSED) -> Bus Creator/4
  Subsystem/1(XMNSEA) -> Bus Creator/1
  G/1 -> Subsystem/1(G)
  Subsystem/8(XMNSEH) -> Bus Creator/8
  Subsystem/3(XMNSEC) -> Bus Creator/3
  Subsystem/7(XMNSEG) -> Bus Creator/7
  Subsystem/9(G_NEW) -> G_NEW/1
  Subsystem/2(XMNSEB) -> Bus Creator/2
  Subsystem/5(XMNSEE) -> Bus Creator/5
  Subsystem/6(XMNSEF) -> Bus Creator/6
  Bus Creator/1 -> Stream 4/1  "Stream 4"

== system COSTEP/Random number generator/Stream Measurements SMEAS Gas analysis1/If Action Subsystem3/Subsystem/Stream 5 ==
  G : Inport
  Bus Creator : BusCreator  Inputs=8
  Subsystem : Subsystem
  Stream 5 : Outport
  G_NEW : Outport  Port=2
  wires:
  Subsystem/4(XMNSED) -> Bus Creator/4
  Subsystem/1(XMNSEA) -> Bus Creator/1
  G/1 -> Subsystem/1(G)
  Subsystem/8(XMNSEH) -> Bus Creator/8
  Subsystem/3(XMNSEC) -> Bus Creator/3
  Subsystem/7(XMNSEG) -> Bus Creator/7
  Subsystem/9(G_NEW) -> G_NEW/1
  Subsystem/2(XMNSEB) -> Bus Creator/2
  Subsystem/5(XMNSEE) -> Bus Creator/5
  Subsystem/6(XMNSEF) -> Bus Creator/6
  Bus Creator/1 -> Stream 5/1  "Stream 5"

== system COSTEP/Random number generator/Stream Measurements SMEAS Gas analysis1/If Action Subsystem3/Subsystem/Stream 6 ==
  G : Inport
  Bus Creator : BusCreator  Inputs=8
  Subsystem : Subsystem
  Stream 6 : Outport
  G_NEW : Outport  Port=2
  wires:
  Subsystem/4(XMNSED) -> Bus Creator/4
  Subsystem/1(XMNSEA) -> Bus Creator/1
  G/1 -> Subsystem/1(G)
  Subsystem/8(XMNSEH) -> Bus Creator/8
  Subsystem/3(XMNSEC) -> Bus Creator/3
  Subsystem/7(XMNSEG) -> Bus Creator/7
  Subsystem/9(G_NEW) -> G_NEW/1
  Subsystem/2(XMNSEB) -> Bus Creator/2
  Subsystem/5(XMNSEE) -> Bus Creator/5
  Subsystem/6(XMNSEF) -> Bus Creator/6
  Bus Creator/1 -> Stream 6/1  "Stream 6"

== system COSTEP/Random number generator/Stream Measurements SMEAS Gas analysis1/If Action Subsystem3/Subsystem/Stream 8 ==
  G : Inport
  Bus Creator : BusCreator  Inputs=8
  Subsystem : Subsystem
  Stream 8 : Outport
  G_NEW : Outport  Port=2
  wires:
  Subsystem/4(XMNSED) -> Bus Creator/4
  Subsystem/1(XMNSEA) -> Bus Creator/1
  G/1 -> Subsystem/1(G)
  Subsystem/8(XMNSEH) -> Bus Creator/8
  Subsystem/3(XMNSEC) -> Bus Creator/3
  Subsystem/7(XMNSEG) -> Bus Creator/7
  Subsystem/9(G_NEW) -> G_NEW/1
  Subsystem/2(XMNSEB) -> Bus Creator/2
  Subsystem/5(XMNSEE) -> Bus Creator/5
  Subsystem/6(XMNSEF) -> Bus Creator/6
  Bus Creator/1 -> Stream 8/1  "Stream 8"

== system COSTEP/Random number generator/Stream Measurements SMEAS Gas analysis1/If Action Subsystem3/Subsystem/Stream 9 ==
  G : Inport
  Bus Creator : BusCreator  Inputs=8
  Subsystem : Subsystem
  Stream 9 : Outport
  G_NEW : Outport  Port=2
  wires:
  Subsystem/4(XMNSED) -> Bus Creator/4
  Subsystem/1(XMNSEA) -> Bus Creator/1
  G/1 -> Subsystem/1(G)
  Subsystem/8(XMNSEH) -> Bus Creator/8
  Subsystem/3(XMNSEC) -> Bus Creator/3
  Subsystem/7(XMNSEG) -> Bus Creator/7
  Subsystem/9(G_NEW) -> G_NEW/1
  Subsystem/2(XMNSEB) -> Bus Creator/2
  Subsystem/5(XMNSEE) -> Bus Creator/5
  Subsystem/6(XMNSEF) -> Bus Creator/6
  Bus Creator/1 -> Stream 9/1  "Stream 9"

== system COSTEP/Random number generator/Stream Measurements SMEAS Product analysis1/Gas Analysis Delay/Subsystem/If Action Subsystem ==
  Action Port : ActionPort  ActionPortLabel=if(u1 == u2)
  Constant : Constant  Value=0
  Out1 : Outport  VectorParamsAs1DForOutWhenUnconnected=off
  wires:
  Constant/1 -> Out1/1

== system COSTEP/Random number generator/Stream Measurements SMEAS Product analysis1/Gas Analysis Delay/Subsystem/If Action Subsystem1 ==
  In1 : Inport
  Action Port : ActionPort  ActionPortLabel=else
  Out1 : Outport  VectorParamsAs1DForOutWhenUnconnected=off
  wires:
  In1/1 -> Out1/1

== system COSTEP/Random number generator/Stream Measurements SMEAS Product analysis1/If Action Subsystem3/Subsystem/Subsystem1 ==
  G : Inport
  Bus Creator : BusCreator  Inputs=5
  Subsystem : Subsystem
  Stream 11 : Outport
  G_NEW : Outport  Port=2
  wires:
  Subsystem/2(XMNSEE) -> Bus Creator/2
  G/1 -> Subsystem/1(G)
  Subsystem/6(G_NEW) -> G_NEW/1
  Subsystem/5(XMNSEH) -> Bus Creator/5
  Subsystem/4(XMNSEG) -> Bus Creator/4
  Subsystem/3(XMNSEF) -> Bus Creator/3
  Subsystem/1(XMNSED) -> Bus Creator/1
  Bus Creator/1 -> Stream 11/1  "Stream 11"

== system COSTEP/Random number generator/Stream Measurements SMEAS Product analysis1/If Action Subsystem3/Subsystem/Subsystem2 ==
  G : Inport
  Bus Creator : BusCreator  Inputs=5
  Subsystem : Subsystem
  Stream 13 : Outport
  G_NEW : Outport  Port=2
  wires:
  Subsystem/2(XMNSEE) -> Bus Creator/2
  G/1 -> Subsystem/1(G)
  Subsystem/6(G_NEW) -> G_NEW/1
  Subsystem/5(XMNSEH) -> Bus Creator/5
  Subsystem/4(XMNSEG) -> Bus Creator/4
  Subsystem/3(XMNSEF) -> Bus Creator/3
  Subsystem/1(XMNSED) -> Bus Creator/1
  Bus Creator/1 -> Stream 13/1  "Stream 13"

== system COSTEP/Reactor/Reaction Rates/Reaction rates lb-mol//h/Reaction rate of reaction 1 lb-mol//ft3·h/If Action Subsystem ==
  In1 : Inport
  Action Port : ActionPort  ActionPortLabel=if( u1>0 & u2>0 )
  Out1 : Outport  VectorParamsAs1DForOutWhenUnconnected=off
  wires:
  In1/1 -> Out1/1

== system COSTEP/Reactor/Reaction Rates/Reaction rates lb-mol//h/Reaction rate of reaction 1 lb-mol//ft3·h/If Action Subsystem2 ==
  In1 : Inport
  Action Port : ActionPort  ActionPortLabel=else
  Out1 : Outport  VectorParamsAs1DForOutWhenUnconnected=off
  wires:
  In1/1 -> Out1/1

== system COSTEP/Reactor/Reaction Rates/Reaction rates lb-mol//h/Reaction rate of reaction 1 lb-mol//ft3·h/RR(1) Reaction rate of 1st reaction lb-mol//ft3·h  ==
  PPR : Inport
  TKR : Inport  Port=2
  "   " : Constant  Value=1.1544
  "    " : Constant  Value=0.3735
  Abs : Abs  SaturateOnIntegerOverflow=off
  Abs1 : Abs  SaturateOnIntegerOverflow=off
  Activation energy cal/mol : Constant  Value=40000
  Bus Selector : BusSelector  OutputSignals=PPR(1),PPR(3),PPR(4)
  Bus Selector1 : BusSelector  OutputSignals=signal1.TESUB8(7)
  Divide : Product  Inputs=*//
  Divide1 : Product  Inputs=4
  Math Function1 : Math  SignedPower=on
  Preexponential factor lb-mol/ft3·h·mmHg : Constant  Value=31.5859536
  Product : Product
  R1F : Math  Operator=pow  SignedPower=on
  R2F : Math  Operator=pow  SignedPower=on
  Subtract : Sum  Inputs=+-
  Universal gas constant cal/mol·K : Constant  Value=1.987
  RR(1) : Outport  VectorParamsAs1DForOutWhenUnconnected=off
  wires:
  "    "/1 -> R2F/2
  Divide/1 -> Subtract/2
  Universal gas constant cal/mol·K/1 -> Divide/2
  "   "/1 -> R1F/2
  Preexponential factor lb-mol/ft3·h·mmHg/1 -> Subtract/1
  Activation energy cal/mol/1 -> Divide/1
  TKR/1 -> Divide/3
  Subtract/1 -> Math Function1/1
  Divide1/1 -> RR(1)/1
  Bus Selector/2 -> Abs1/1  "<PPR(3)>"
  Abs/1 -> R1F/1
  Abs1/1 -> R2F/1
  PPR/1 -> Bus Selector/1
  Bus Selector/1 -> Abs/1  "<PPR(1)>"
  R1F/1 -> Divide1/2
  R2F/1 -> Divide1/3
  Bus Selector/3 -> Divide1/4  "<PPR(4)>"
  [TESUB8] -> Bus Selector1/1
  Math Function1/1 -> Product/1
  Bus Selector1/1 -> Product/2  "<TESUB8(7)>"
  Product/1 -> Divide1/1

== system COSTEP/Reactor/Reaction Rates/Reaction rates lb-mol//h/Reaction rate of reaction 2 lb-mol//ft3·h/If Action Subsystem ==
  In1 : Inport
  Action Port : ActionPort  ActionPortLabel=if( u1>0 & u2>0)
  Out1 : Outport  VectorParamsAs1DForOutWhenUnconnected=off
  wires:
  In1/1 -> Out1/1

== system COSTEP/Reactor/Reaction Rates/Reaction rates lb-mol//h/Reaction rate of reaction 2 lb-mol//ft3·h/If Action Subsystem2 ==
  In1 : Inport
  Action Port : ActionPort  ActionPortLabel=else
  Out1 : Outport  VectorParamsAs1DForOutWhenUnconnected=off
  wires:
  In1/1 -> Out1/1

== system COSTEP/Reactor/Reaction Rates/Reaction rates lb-mol//h/Reaction rate of reaction 2 lb-mol//ft3·h/RR(2) Reaction rate of 2nd reaction lb-mol//ft3·h  ==
  PPR : Inport
  TKR : Inport  Port=2
  "   " : Constant  Value=1.1544
  "    " : Constant  Value=0.3735
  Abs : Abs  SaturateOnIntegerOverflow=off
  Abs1 : Abs  SaturateOnIntegerOverflow=off
  Activation energy cal/mol : Constant  Value=20000
  Bus Selector : BusSelector  OutputSignals=PPR(1),PPR(3),PPR(5)
  Bus Selector1 : BusSelector  OutputSignals=signal1.TESUB8(8)
  Divide : Product  Inputs=*//
  Divide1 : Product  Inputs=4
  Math Function2 : Math  SignedPower=on
  Preexponential factor lb-mol/ft3·h·mmHg : Constant  Value=3.00094014
  Product : Product
  R1F : Math  Operator=pow  SignedPower=on
  R2F : Math  Operator=pow  SignedPower=on
  Subtract : Sum  Inputs=+-
  Universal gas constant cal/mol·K : Constant  Value=1.987
  RR(2) : Outport  VectorParamsAs1DForOutWhenUnconnected=off
  wires:
  "    "/1 -> R2F/2
  Divide/1 -> Subtract/2
  Universal gas constant cal/mol·K/1 -> Divide/2
  "   "/1 -> R1F/2
  Preexponential factor lb-mol/ft3·h·mmHg/1 -> Subtract/1
  Activation energy cal/mol/1 -> Divide/1
  TKR/1 -> Divide/3
  Subtract/1 -> Math Function2/1
  Divide1/1 -> RR(2)/1
  Bus Selector/2 -> Abs1/1  "<PPR(3)>"
  Abs/1 -> R1F/1
  Abs1/1 -> R2F/1
  PPR/1 -> Bus Selector/1
  Bus Selector/1 -> Abs/1  "<PPR(1)>"
  R1F/1 -> Divide1/2
  R2F/1 -> Divide1/3
  Bus Selector/3 -> Divide1/4  "<PPR(5)>"
  [TESUB8] -> Bus Selector1/1
  Product/1 -> Divide1/1
  Math Function2/1 -> Product/1
  Bus Selector1/1 -> Product/2  "<TESUB8(8)>"

== system COSTEP/Reactor/Reactor Heat exchanger/Reactor Heat exchanger/Cooling water outlet temperature/TCWR Inlet temperature of cooling water °C  ==
  Add : Sum
  Bus Selector : BusSelector  OutputSignals=signal1.TESUB8(5)
  Bus Selector1 : BusSelector  OutputSignals=IDV(4)
  Constant : Constant  Value=5
  Product1 : Product
  TCWR : Outport  VectorParamsAs1DForOutWhenUnconnected=off
  wires:
  Constant/1 -> Product1/2
  Bus Selector/1 -> Add/1  "<TESUB8(5)>"
  Bus Selector1/1 -> Product1/1  "<IDV(4)>"
  [TESUB8] -> Bus Selector/1
  Product1/1 -> Add/2
  [IDV] -> Bus Selector1/1
  Add/1 -> TCWR/1

== system COSTEP/Reactor/Reactor Heat exchanger/Reactor Heat exchanger/Subsystem/If Action Subsystem ==
  In1 : Inport
  Action Port : ActionPort  ActionPortLabel=if(u1 > 50)
  Out1 : Outport  VectorParamsAs1DForOutWhenUnconnected=off
  wires:
  In1/1 -> Out1/1

== system COSTEP/Reactor/Reactor Heat exchanger/Reactor Heat exchanger/Subsystem/If Action Subsystem1 ==
  In1 : Inport
  Action Port : ActionPort  ActionPortLabel=elseif(u1 < 10)
  Out1 : Outport  VectorParamsAs1DForOutWhenUnconnected=off
  wires:
  In1/1 -> Out1/1

== system COSTEP/Reactor/Reactor Heat exchanger/Reactor Heat exchanger/Subsystem/If Action Subsystem2 ==
  In1 : Inport
  Action Port : ActionPort  ActionPortLabel=else
  Out1 : Outport  VectorParamsAs1DForOutWhenUnconnected=off
  wires:
  In1/1 -> Out1/1

== system COSTEP/Separator/Stream 9/Subsystem/Pressure drop/If Action Subsystem ==
  In1 : Inport
  Action Port : ActionPort  ActionPortLabel=if(u1 < 0)
  Out1 : Outport  VectorParamsAs1DForOutWhenUnconnected=off
  wires:
  In1/1 -> Out1/1

== system COSTEP/Separator/Stream 9/Subsystem/Pressure drop/If Action Subsystem1 ==
  In1 : Inport
  Action Port : ActionPort  ActionPortLabel=else
  Out1 : Outport  VectorParamsAs1DForOutWhenUnconnected=off
  wires:
  In1/1 -> Out1/1

== system COSTEP/Stream Measurements/Subsystem6/A and C feed stream/Composition measurement mol%/Subsystem ==
  XST : Inport
  XMNSE : Inport  Port=2
  Bus Selector : BusSelector  OutputSignals=XMNSEA,XMNSEB,XMNSEC
  Process Noise I=23-1 : mylib/Process Noise I=23-36  SystemSampleTime=-1  VariantActivationTime=update diagram  AllowFlexibleInterface=on  Latency=0  AutoFrameSizeCalculation=off
  Process Noise I=23-2 : mylib/Process Noise I=23-36  SystemSampleTime=-1  VariantActivationTime=update diagram  AllowFlexibleInterface=on  Latency=0  AutoFrameSizeCalculation=off
  Process Noise I=23-36 : mylib/Process Noise I=23-36  SystemSampleTime=-1  VariantActivationTime=update diagram  AllowFlexibleInterface=on  Latency=0  AutoFrameSizeCalculation=off
  Subsystem : Subsystem
  SMEASXA(4) : Outport  VectorParamsAs1DForOutWhenUnconnected=off
  SMEASXB(4) : Outport  Port=2  VectorParamsAs1DForOutWhenUnconnected=off
  SMEASXC(4) : Outport  Port=3  VectorParamsAs1DForOutWhenUnconnected=off
  wires:
  Process Noise I=23-36/1 -> SMEASXA(4)/1
  Process Noise I=23-1/1 -> SMEASXB(4)/1
  Bus Selector/2 -> Process Noise I=23-1/2  "<XMNSEB>"
  Process Noise I=23-2/1 -> SMEASXC(4)/1
  Bus Selector/3 -> Process Noise I=23-2/2  "<XMNSEC>"
  Bus Selector/1 -> Process Noise I=23-36/2  "<XMNSEA>"
  XST/1 -> Subsystem/1(XST)
  Subsystem/1(XCMPA) -> Process Noise I=23-36/1
  Subsystem/2(XCMPB) -> Process Noise I=23-1/1
  Subsystem/3(XCMPC) -> Process Noise I=23-2/1
  XMNSE/1 -> Bus Selector/1

== system COSTEP/Stream Measurements/Subsystem6/A and C feed stream/Flow measurement in kg//h/XMWS Molecular weight of Stream lb//lb-mol ==
  XST : Inport
  Product : Product
  Sum of Elements : Sum  Inputs=+
  "XMW(I) Molecular weight of components lb/lb-mol " : Constant  Value=XMW
  XMWS : Outport  VectorParamsAs1DForOutWhenUnconnected=off
  wires:
  Sum of Elements/1 -> XMWS/1
  Product/1 -> Sum of Elements/1
  XST/1 -> Product/1
  "XMW(I) Molecular weight of components lb/lb-mol "/1 -> Product/2

== system COSTEP/Stream Measurements/Subsystem6/A feed stream/Composition measurement mol%/Subsystem ==
  XST : Inport
  XMNSE : Inport  Port=2
  Bus Selector : BusSelector  OutputSignals=XMNSEA,XMNSEB
  Process Noise I=23-1 : mylib/Process Noise I=23-36  SystemSampleTime=-1  VariantActivationTime=update diagram  AllowFlexibleInterface=on  Latency=0  AutoFrameSizeCalculation=off
  Process Noise I=23-36 : mylib/Process Noise I=23-36  SystemSampleTime=-1  VariantActivationTime=update diagram  AllowFlexibleInterface=on  Latency=0  AutoFrameSizeCalculation=off
  Subsystem : Subsystem
  SMEASXA(1) : Outport  VectorParamsAs1DForOutWhenUnconnected=off
  SMEASXB(1) : Outport  Port=2  VectorParamsAs1DForOutWhenUnconnected=off
  wires:
  Process Noise I=23-36/1 -> SMEASXA(1)/1
  Process Noise I=23-1/1 -> SMEASXB(1)/1
  Bus Selector/2 -> Process Noise I=23-1/2  "<XMNSEB>"
  Bus Selector/1 -> Process Noise I=23-36/2  "<XMNSEA>"
  XST/1 -> Subsystem/1(XST)
  Subsystem/1(XCMPA) -> Process Noise I=23-36/1
  Subsystem/2(XCMPB) -> Process Noise I=23-1/1
  XMNSE/1 -> Bus Selector/1

== system COSTEP/Stream Measurements/Subsystem6/A feed stream/Flow measurement in kg//h/XMWS Molecular weight of Stream lb//lb-mol ==
  XST : Inport
  Product : Product
  Sum of Elements : Sum  Inputs=+
  "XMW(I) Molecular weight of components lb/lb-mol " : Constant  Value=XMW
  XMWS : Outport  VectorParamsAs1DForOutWhenUnconnected=off
  wires:
  Sum of Elements/1 -> XMWS/1
  Product/1 -> Sum of Elements/1
  XST/1 -> Product/1
  "XMW(I) Molecular weight of components lb/lb-mol "/1 -> Product/2

== system COSTEP/Stream Measurements/Subsystem6/Condenser product stream/Composition measurement mol%/Subsystem ==
  XST : Inport
  XMNSE : Inport  Port=2
  Bus Selector : BusSelector  OutputSignals=XMNSEA,XMNSEB,XMNSEC,XMNSED,XMNSEE,XMNSEF,XMNSEG,XMNSEH
  Process Noise I=23-{1..7,36} (8 alike) : mylib/Process Noise I=23-36  SystemSampleTime=-1  VariantActivationTime=update diagram  AllowFlexibleInterface=on  Latency=0  AutoFrameSizeCalculation=off
  Subsystem : Subsystem
  SMEASXA : Outport  VectorParamsAs1DForOutWhenUnconnected=off
  SMEASXB : Outport  Port=2  VectorParamsAs1DForOutWhenUnconnected=off
  SMEASXC : Outport  Port=3  VectorParamsAs1DForOutWhenUnconnected=off
  SMEASXD : Outport  Port=4  VectorParamsAs1DForOutWhenUnconnected=off
  SMEASXE : Outport  Port=5  VectorParamsAs1DForOutWhenUnconnected=off
  SMEASXF : Outport  Port=6  VectorParamsAs1DForOutWhenUnconnected=off
  SMEASXG : Outport  Port=7  VectorParamsAs1DForOutWhenUnconnected=off
  SMEASXH : Outport  Port=8  VectorParamsAs1DForOutWhenUnconnected=off
  wires:
  Process Noise I=23-36/1 -> SMEASXA/1
  Process Noise I=23-1/1 -> SMEASXB/1
  Bus Selector/2 -> Process Noise I=23-1/2  "<XMNSEB>"
  Process Noise I=23-2/1 -> SMEASXC/1
  Process Noise I=23-3/1 -> SMEASXD/1
  Process Noise I=23-4/1 -> SMEASXE/1
  Process Noise I=23-5/1 -> SMEASXF/1
  Process Noise I=23-6/1 -> SMEASXG/1
  Process Noise I=23-7/1 -> SMEASXH/1
  Bus Selector/7 -> Process Noise I=23-6/2  "<XMNSEG>"
  Bus Selector/8 -> Process Noise I=23-7/2  "<XMNSEH>"
  Bus Selector/6 -> Process Noise I=23-5/2  "<XMNSEF>"
  Bus Selector/5 -> Process Noise I=23-4/2  "<XMNSEE>"
  Bus Selector/4 -> Process Noise I=23-3/2  "<XMNSED>"
  Bus Selector/3 -> Process Noise I=23-2/2  "<XMNSEC>"
  Bus Selector/1 -> Process Noise I=23-36/2  "<XMNSEA>"
  XST/1 -> Subsystem/1(XST)
  Subsystem/1(XCMPA) -> Process Noise I=23-36/1
  Subsystem/2(XCMPB) -> Process Noise I=23-1/1
  Subsystem/3(XCMPC) -> Process Noise I=23-2/1
  Subsystem/4(XCMPD) -> Process Noise I=23-3/1
  Subsystem/5("XCMPE ") -> Process Noise I=23-4/1
  Subsystem/6("XCMPF ") -> Process Noise I=23-5/1
  Subsystem/7(XCMPG) -> Process Noise I=23-6/1
  Subsystem/8("XCMPH ") -> Process Noise I=23-7/1
  XMNSE/1 -> Bus Selector/1

== system COSTEP/Stream Measurements/Subsystem6/Condenser product stream/Flow measurement in kg//h/XMWS Molecular weight of Stream lb//lb-mol ==
  XST : Inport
  Product : Product
  Sum of Elements : Sum  Inputs=+
  "XMW(I) Molecular weight of components lb/lb-mol " : Constant  Value=XMW
  XMWS : Outport  VectorParamsAs1DForOutWhenUnconnected=off
  wires:
  Sum of Elements/1 -> XMWS/1
  Product/1 -> Sum of Elements/1
  XST/1 -> Product/1
  "XMW(I) Molecular weight of components lb/lb-mol "/1 -> Product/2
